simulink model "Copy_of_CoupledTanks_WCPS_v2_DoubleSD"  (Simulink 8.1)
settings: Solver=ode4  StartTime=0.0  StopTime=Tf  FixedStep=0.2  RelTol=1e-3
values from neighbouring files (symbols this model uses):
  A1 = 0.06    [Copy_of_CoupledTanks_WCPS_2_DoublePS.m]    (also in CoupledTanks_WCPS_2_DoublePS.m; DoublePlant_PS_INI3_RSSI74_1.mat; Wireless_74_Initial_98.mat)
  A2 = 0.3    [Copy_of_CoupledTanks_WCPS_2_DoublePS.m]    (also in CoupledTanks_WCPS_2_DoublePS.m; DoublePlant_PS_INI3_RSSI74_1.mat; Wireless_74_Initial_98.mat)
  alpha1 = 10    [Copy_of_CoupledTanks_WCPS_2_DoublePS.m]    (also in CoupledTanks_WCPS_2_DoublePS.m; DoublePlant_PS_INI3_RSSI74_1.mat; Wireless_74_Initial_98.mat)
  AR = 0.3    [Copy_of_CoupledTanks_WCPS_2_DoublePS.m]    (also in CoupledTanks_WCPS_2_DoublePS.m; DoublePlant_PS_INI3_RSSI74_1.mat; Wireless_74_Initial_98.mat)
  delta_t = 1    [Copy_of_CoupledTanks_WCPS_2_DoublePS.m]    (also in CoupledTanks_WCPS_2_DoublePS.m = 0.2; DoublePlant_PS_INI3_RSSI74_1.mat; Wireless_74_Initial_98.mat = 0.25)
  EMPeriod = 1    [Copy_of_CoupledTanks_WCPS_2_DoublePS.m]    (also in CoupledTanks_WCPS_2_DoublePS.m; DoublePlant_PS_INI3_RSSI74_1.mat; Wireless_74_Initial_98.mat = 8)
  g = 9.8    [Copy_of_CoupledTanks_WCPS_2_DoublePS.m]    (also in CoupledTanks_WCPS_2_DoublePS.m; DoublePlant_PS_INI3_RSSI74_1.mat; Wireless_74_Initial_98.mat)
  kd = 0    [Copy_of_CoupledTanks_WCPS_2_DoublePS.m]    (also in CoupledTanks_WCPS_2_DoublePS.m; DoublePlant_PS_INI3_RSSI74_1.mat; Wireless_74_Initial_98.mat)
  ki = 0.5    [Copy_of_CoupledTanks_WCPS_2_DoublePS.m]    (also in CoupledTanks_WCPS_2_DoublePS.m; DoublePlant_PS_INI3_RSSI74_1.mat; Wireless_74_Initial_98.mat)
  kp = 5    [Copy_of_CoupledTanks_WCPS_2_DoublePS.m]    (also in CoupledTanks_WCPS_2_DoublePS.m; DoublePlant_PS_INI3_RSSI74_1.mat; Wireless_74_Initial_98.mat)
  L1H = 9    [Copy_of_CoupledTanks_WCPS_2_DoublePS.m]    (also in CoupledTanks_WCPS_2_DoublePS.m = 90; DoublePlant_PS_INI3_RSSI74_1.mat; Wireless_74_Initial_98.mat)
  L1ini = 9    [Copy_of_CoupledTanks_WCPS_2_DoublePS.m]    (also in CoupledTanks_WCPS_2_DoublePS.m; DoublePlant_PS_INI3_RSSI74_1.mat; Wireless_74_Initial_98.mat = 8.14638203104)
  L1up = 10    [Copy_of_CoupledTanks_WCPS_2_DoublePS.m]    (also in CoupledTanks_WCPS_2_DoublePS.m; DoublePlant_PS_INI3_RSSI74_1.mat; Wireless_74_Initial_98.mat)
  L2H = 11.5    [Copy_of_CoupledTanks_WCPS_2_DoublePS.m]    (also in CoupledTanks_WCPS_2_DoublePS.m = 115; DoublePlant_PS_INI3_RSSI74_1.mat; Wireless_74_Initial_98.mat)
  L2ini = 9.15    [Copy_of_CoupledTanks_WCPS_2_DoublePS.m]    (also in CoupledTanks_WCPS_2_DoublePS.m; DoublePlant_PS_INI3_RSSI74_1.mat; Wireless_74_Initial_98.mat = 6.34545311751)
  L2sp = 11.05    [Copy_of_CoupledTanks_WCPS_2_DoublePS.m]    (also in CoupledTanks_WCPS_2_DoublePS.m; DoublePlant_PS_INI3_RSSI74_1.mat; Wireless_74_Initial_98.mat)
  L2up = 13    [Copy_of_CoupledTanks_WCPS_2_DoublePS.m]    (also in CoupledTanks_WCPS_2_DoublePS.m; DoublePlant_PS_INI3_RSSI74_1.mat; Wireless_74_Initial_98.mat)
  LRdown = 0    [Copy_of_CoupledTanks_WCPS_2_DoublePS.m]    (also in CoupledTanks_WCPS_2_DoublePS.m; DoublePlant_PS_INI3_RSSI74_1.mat; Wireless_74_Initial_98.mat)
  LRH = 5.7    [Copy_of_CoupledTanks_WCPS_2_DoublePS.m]    (also in CoupledTanks_WCPS_2_DoublePS.m = 57; DoublePlant_PS_INI3_RSSI74_1.mat; Wireless_74_Initial_98.mat)
  LRini = 5.65    [Copy_of_CoupledTanks_WCPS_2_DoublePS.m]    (also in CoupledTanks_WCPS_2_DoublePS.m; DoublePlant_PS_INI3_RSSI74_1.mat; Wireless_74_Initial_98.mat = 4.28399951136)
  LRL = 0.2    [Copy_of_CoupledTanks_WCPS_2_DoublePS.m]    (also in CoupledTanks_WCPS_2_DoublePS.m = 0; DoublePlant_PS_INI3_RSSI74_1.mat; Wireless_74_Initial_98.mat)
  LRup = 9    [Copy_of_CoupledTanks_WCPS_2_DoublePS.m]    (also in CoupledTanks_WCPS_2_DoublePS.m; DoublePlant_PS_INI3_RSSI74_1.mat; Wireless_74_Initial_98.mat)
  p12 = 1    [Copy_of_CoupledTanks_WCPS_2_DoublePS.m]    (also in CoupledTanks_WCPS_2_DoublePS.m; DoublePlant_PS_INI3_RSSI74_1.mat; Wireless_74_Initial_98.mat)
  p22 = 1    [Copy_of_CoupledTanks_WCPS_2_DoublePS.m]    (also in CoupledTanks_WCPS_2_DoublePS.m; DoublePlant_PS_INI3_RSSI74_1.mat; Wireless_74_Initial_98.mat)
  p2tap = 1    [Copy_of_CoupledTanks_WCPS_2_DoublePS.m]    (also in CoupledTanks_WCPS_2_DoublePS.m; DoublePlant_PS_INI3_RSSI74_1.mat; Wireless_74_Initial_98.mat)
  PumpMAX = 60    [Copy_of_CoupledTanks_WCPS_2_DoublePS.m]    (also in CoupledTanks_WCPS_2_DoublePS.m; DoublePlant_PS_INI3_RSSI74_1.mat; Wireless_74_Initial_98.mat)
  R1 = 0.0005    [Copy_of_CoupledTanks_WCPS_2_DoublePS.m]    (also in CoupledTanks_WCPS_2_DoublePS.m; DoublePlant_PS_INI3_RSSI74_1.mat; Wireless_74_Initial_98.mat)
  R1tap = 0.001    [Copy_of_CoupledTanks_WCPS_2_DoublePS.m]    (also in CoupledTanks_WCPS_2_DoublePS.m; DoublePlant_PS_INI3_RSSI74_1.mat; Wireless_74_Initial_98.mat)
  R2 = 0.001    [Copy_of_CoupledTanks_WCPS_2_DoublePS.m]    (also in CoupledTanks_WCPS_2_DoublePS.m; DoublePlant_PS_INI3_RSSI74_1.mat; Wireless_74_Initial_98.mat)
  rho = 1000    [Copy_of_CoupledTanks_WCPS_2_DoublePS.m]    (also in CoupledTanks_WCPS_2_DoublePS.m; DoublePlant_PS_INI3_RSSI74_1.mat; Wireless_74_Initial_98.mat)
settings Model: Creator=Rhine  LastModifiedBy=sywxh2012
settings DebuggingCC: MultiTaskDSMMsg=none  MultiTaskRateTransMsg=warning

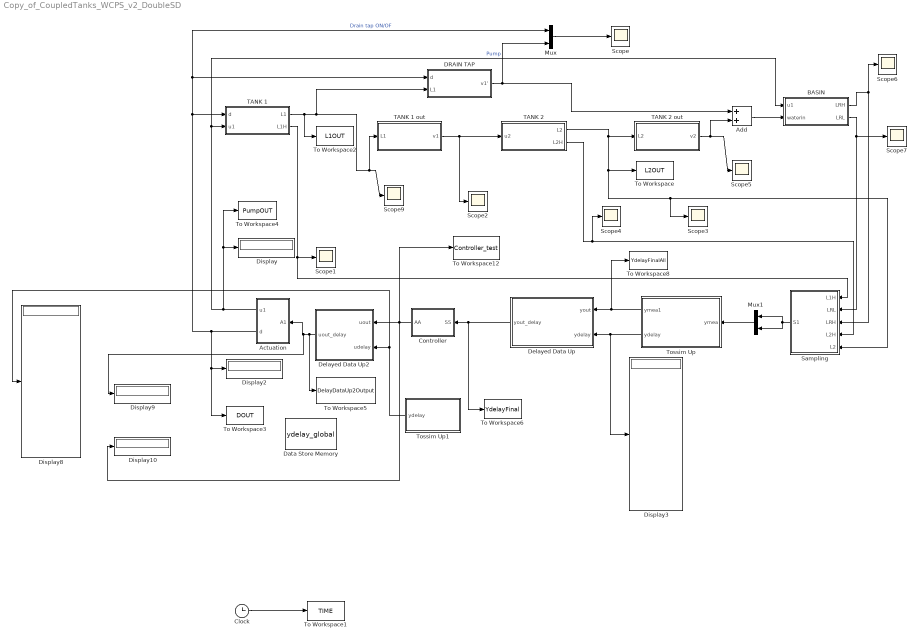
== system Copy_of_CoupledTanks_WCPS_v2_DoubleSD ==
  Actuation : Subsystem
  Add : Sum
  BASIN : Subsystem
  Clock : Clock
  Controller : Subsystem
  DRAIN TAP : Subsystem
  Data Store Memory : DataStoreMemory  DataStoreName=ydelay_global  ReadBeforeWriteMsg=warning  WriteAfterWriteMsg=warning  WriteAfterReadMsg=warning  InitialValue=[1; 1; 1; 1; 1; 1; 1; 1; 1; 1; 1; 1; 1; 1; 1]  OutDataTypeStr=uint32
  Delayed Data Up : MATLAB Function  TreatAsAtomicUnit=on
  Delayed Data Up2 : MATLAB Function  TreatAsAtomicUnit=on
  Display{,2..3,8..10} (6 alike) : Display
  Mux : Mux  Inputs=2
  Mux1 : Mux  Inputs=2
  Sampling : Subsystem
  Scope{,1..7,9} (9 alike) : Scope
      Scope2 settings: SaveName=ScopeData2
      Scope3 settings: SaveName=ScopeData15
      Scope4 settings: SaveName=ScopeData4
      Scope5 settings: SaveName=ScopeData5
      Scope6 settings: SaveName=ScopeData7
      Scope7 settings: SaveName=ScopeData8
      Scope9 settings: YMin=7.45104  YMax=8.23536  SaveName=ScopeData10
  TANK 1 : Subsystem
  TANK 1 out : Subsystem
  TANK 2 : Subsystem
  TANK 2 out : Subsystem
  To Workspace : ToWorkspace  VariableName=L2OUT  SampleTime=-1
  To Workspace1 : ToWorkspace  VariableName=TIME  SampleTime=-1
  To Workspace12 : ToWorkspace  VariableName=Controller_test  SampleTime=-1
  To Workspace2 : ToWorkspace  VariableName=L1OUT  SampleTime=-1
  To Workspace3 : ToWorkspace  VariableName=DOUT  SampleTime=-1
  To Workspace4 : ToWorkspace  VariableName=PumpOUT  SampleTime=-1
  To Workspace5 : ToWorkspace  VariableName=DelayDataUp2Output  SampleTime=-1
  To Workspace6 : ToWorkspace  VariableName=YdelayFinal  SampleTime=-1
  To Workspace8 : ToWorkspace  VariableName=YdelayFinalAll  SampleTime=-1
  Tossim Up : MATLAB Function  TreatAsAtomicUnit=on
  Tossim Up1 : MATLAB Function  TreatAsAtomicUnit=on
  wires:
  TANK 1/1(L1) -> DRAIN TAP/2(L1), TANK 1 out/1(L1), Scope9/1, To Workspace2/1
  TANK 2/1(L2) -> TANK 2 out/1(L2), To Workspace/1, Scope3/1, Sampling/5(L2)
  DRAIN TAP/1(v1') -> Add/1, Mux/2
  TANK 2 out/1(v2) -> Scope5/1, Add/2
  TANK 1/2(L1H) -> Scope1/1, Sampling/1(L1H)
  TANK 1 out/1(v1) -> TANK 2/1(u2), Scope2/1
  TANK 2/2(L2H) -> Scope4/1, Sampling/4(L2H)
  Add/1 -> BASIN/2(waterin)
  BASIN/1(LRH) -> Scope6/1, Sampling/3(LRH)
  BASIN/2(LRL) -> Scope7/1, Sampling/2(LRL)
  Actuation/1(u1) -> Display/1, To Workspace4/1, TANK 1/2(u1), BASIN/1(u1)  "Pump"
  Actuation/2(d) -> TANK 1/1(d), DRAIN TAP/1(d), Mux/1, Display2/1, To Workspace3/1  "Drain tap ON/OF"
  Clock/1 -> To Workspace1/1
  Mux/1 -> Scope/1
  Tossim Up/1(ymea1) -> Delayed Data Up/1(yout), To Workspace8/1
  Tossim Up/2(ydelay) -> Display3/1, Delayed Data Up/2(ydelay)
  Sampling/1(S1) -> Mux1/2, Mux1/1
  Mux1/1 -> Tossim Up/1(ymea)
  Controller/1(AA) -> To Workspace12/1, Display10/1, Delayed Data Up2/1(uout)
  Delayed Data Up2/1(uout_delay) -> To Workspace5/1, Display9/1, Actuation/1(A1)
  Tossim Up1/1(ydelay) -> Display8/1, Delayed Data Up2/2(udelay)
  Delayed Data Up/1(yout_delay) -> To Workspace6/1, Controller/1(SS)

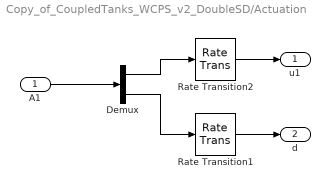
== system Copy_of_CoupledTanks_WCPS_v2_DoubleSD/Actuation ==
  A1 : Inport
  Demux : Demux  Outputs=2
  Rate Transition1 : RateTransition  OutPortSampleTime=delta_t
  Rate Transition2 : RateTransition  OutPortSampleTime=delta_t
  u1 : Outport
  d : Outport  Port=2
  wires:
  A1/1 -> Demux/1
  Rate Transition2/1 -> u1/1
  Rate Transition1/1 -> d/1
  Demux/1 -> Rate Transition2/1
  Demux/2 -> Rate Transition1/1

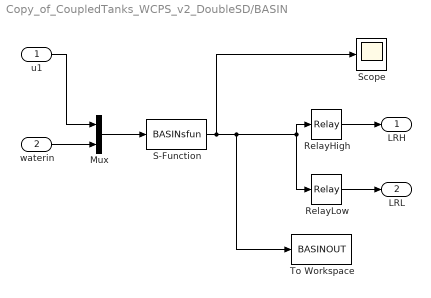
== system Copy_of_CoupledTanks_WCPS_v2_DoubleSD/BASIN ==
  u1 : Inport
  waterin : Inport  Port=2
  Mux : Mux  Inputs=2
  RelayHigh : Relay  OnSwitchValue=LRH  OffSwitchValue=LRH
  RelayLow : Relay  OnSwitchValue=LRL  OffSwitchValue=LRL  OnOutputValue=0  OffOutputValue=1
  S-Function : S-Function  FunctionName=BASINsfun  Parameters=alpha1,AR,LRup,LRdown,rho,LRini  EnableBusSupport=off
  Scope : Scope
      settings: SaveName=ScopeData6
  To Workspace : ToWorkspace  VariableName=BASINOUT  SampleTime=-1
  LRH : Outport
  LRL : Outport  Port=2
  wires:
  RelayLow/1 -> LRL/1
  RelayHigh/1 -> LRH/1
  S-Function/1 -> RelayHigh/1, RelayLow/1, To Workspace/1, Scope/1
  u1/1 -> Mux/1
  waterin/1 -> Mux/2
  Mux/1 -> S-Function/1

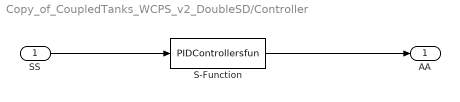
== system Copy_of_CoupledTanks_WCPS_v2_DoubleSD/Controller ==
  SS : Inport
  S-Function : S-Function  FunctionName=PIDControllersfun  Parameters=L2sp,kp,ki,kd,PumpMAX,delta_t,EMPeriod,L2ini  EnableBusSupport=off
  AA : Outport
  wires:
  SS/1 -> S-Function/1
  S-Function/1 -> AA/1

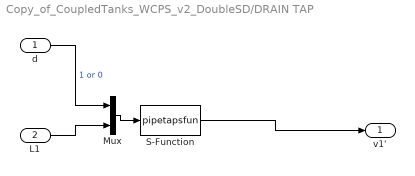
== system Copy_of_CoupledTanks_WCPS_v2_DoubleSD/DRAIN TAP ==
  d : Inport
  L1 : Inport  Port=2
  Mux : Mux  Inputs=2
  S-Function : S-Function  FunctionName=pipetapsfun  Parameters=rho,R1tap,p2tap,g  EnableBusSupport=off
  v1' : Outport
  wires:
  d/1 -> Mux/1  "1 or 0"
  L1/1 -> Mux/2
  Mux/1 -> S-Function/1
  S-Function/1 -> v1'/1

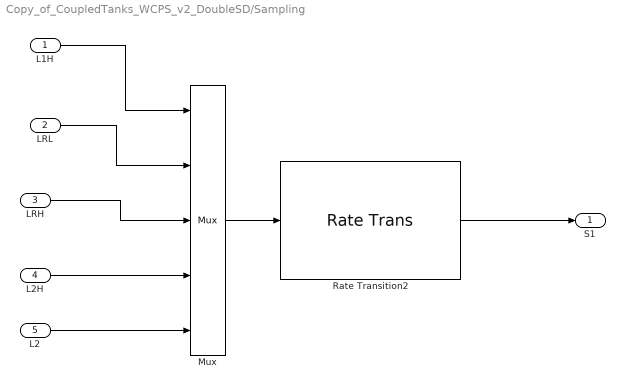
== system Copy_of_CoupledTanks_WCPS_v2_DoubleSD/Sampling ==
  L1H : Inport
  LRL : Inport  Port=2
  LRH : Inport  Port=3
  L2H : Inport  Port=4
  L2 : Inport  Port=5
  Mux : Mux  Inputs=5
  Rate Transition2 : RateTransition  OutPortSampleTime=delta_t
  S1 : Outport
  wires:
  Mux/1 -> Rate Transition2/1
  L1H/1 -> Mux/1
  LRL/1 -> Mux/2
  LRH/1 -> Mux/3
  L2H/1 -> Mux/4
  L2/1 -> Mux/5
  Rate Transition2/1 -> S1/1

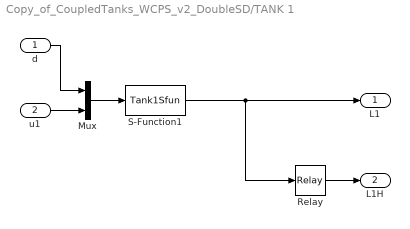
== system Copy_of_CoupledTanks_WCPS_v2_DoubleSD/TANK 1 ==
  d : Inport
  u1 : Inport  Port=2
  Mux : Mux  Inputs=2
  Relay : Relay  OnSwitchValue=L1H  OffSwitchValue=L1H
  S-Function1 : S-Function  FunctionName=Tank1Sfun  Parameters=A1,L1up,rho,alpha1,R1,p12,R1tap,p2tap,g,L1ini  EnableBusSupport=off
  L1 : Outport
  L1H : Outport  Port=2
  wires:
  Relay/1 -> L1H/1
  S-Function1/1 -> L1/1, Relay/1
  d/1 -> Mux/1
  u1/1 -> Mux/2
  Mux/1 -> S-Function1/1

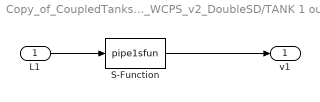
== system Copy_of_CoupledTanks_WCPS_v2_DoubleSD/TANK 1 out ==
  L1 : Inport
  S-Function : S-Function  FunctionName=pipe1sfun  Parameters=rho,R1,p12,g  EnableBusSupport=off
  v1 : Outport
  wires:
  L1/1 -> S-Function/1
  S-Function/1 -> v1/1

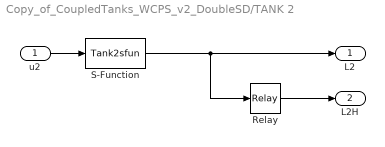
== system Copy_of_CoupledTanks_WCPS_v2_DoubleSD/TANK 2 ==
  u2 : Inport
  Relay : Relay  OnSwitchValue=L2H  OffSwitchValue=L2H
  S-Function : S-Function  FunctionName=Tank2sfun  Parameters=A2,L2up,rho,R2,p22,g,L2ini  EnableBusSupport=off
  L2 : Outport
  L2H : Outport  Port=2
  wires:
  Relay/1 -> L2H/1
  u2/1 -> S-Function/1
  S-Function/1 -> L2/1, Relay/1

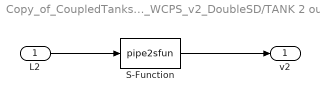
== system Copy_of_CoupledTanks_WCPS_v2_DoubleSD/TANK 2 out ==
  L2 : Inport
  S-Function : S-Function  FunctionName=pipe2sfun  Parameters=rho,R2,p22,g  EnableBusSupport=off
  v2 : Outport
  wires:
  L2/1 -> S-Function/1
  S-Function/1 -> v2/1

== matlab function Tossim Up ==
  data: ymea1 output double; ymea input double; ydelay output double; ydelay_global data_store_memory double
function [ymea1, ydelay]  = Tossim_block(ymea)
% Inputs:
% ymea: measurement from structure
% Outputs:
% ymea1: measurement output
% ydelay: delay traces
persistent delay1 % delay trace
persistent i  % count
persistent last_emergency_instance RetransCounter
global ydelay_global


% allow these matlab functions to be used in Embedded Matlab block
eml.extrinsic('python');
eml.extrinsic('num2str');
eml.extrinsic('str2num');
eml.extrinsic('delay_summary');
eml.extrinsic('disp');
eml.extrinsic('ps_aggregation');
eml.extrinsic('for');
eml.extrinsic('end');

if isempty(i)
    i = 0;
end

ydelay = [1 0 0 0 0 0 0 0 0 0 0 0 0 0 0]'; %No, delay of L1H, delay of L2H, delay of L2, delay of LRL, delay of LRH delay of L1H, delay of L2H, delay of L2, delay of LRL, delay of LRH
% call python to communicate with TOSSIM
emergency_instance=ymea'

%below created in iccps15
%call_count = 55; % number of slots + 1 for PS(i.e., number of client calls made + 1) per TDMA schedule, +1 to have full 53 slots executed
call_count = 49; % number of slots + 1 for Slote Stealing(i.e., number of client calls made + 1) per TDMA schedule, +1 to have full 53 slots executed

rssi = -74;%below is where we inject the senosor status into TOSSIM

[resultz] = ps_aggregation(call_count, rssi, emergency_instance);

end_to_end_delivery_result_aggregated = sum(resultz)
[delay] = delay_summary(end_to_end_delivery_result_aggregated);

delay

% assign delay
ydelay = delay';

last_emergency_instance=ymea';
delay1 = ydelay;
i = i+1;

ymea1 = [0 0 0 0 0 0 0 0 0 0]'; %two plants, 10 sensors
ymea1 = ymea;

for i_yg = 1:15
    ydelay_global(i_yg, 1) = ydelay(i_yg, 1);
end

% disp('Plant 1, TOSSIM Uplink Block, is called');

== matlab function Delayed Data Up ==
  data: yout input double; ydelay input double; yout_delay output double; structure parameter double
function yout_delay   = delay_block(yout,ydelay, structure)

% Inputs: 
% yout: measurements output
% ydelay: delay traces
% structure: other necessary information 
% Inputs: 
% yout: measurements output
% ydelay: delay traces

% Outputs:
% yout_delay: delayed measurements output for controller
persistent  i yin_d 
persistent yin delay yin_all num
eml.extrinsic('disp');

sennum=5;  %number of the sensors
step_count=100000; %step_count

% initialize parameters
if isempty(yin)
    i = structure.i;
    yin = structure.yin;
    yin_d = structure.yin_d; 
    yin_all = zeros(step_count+1,5); %zeros (step count, sensor number)
    
    delay = zeros(1,5+1);         %initialized
    delay = ydelay';
    
    num = 0;
end

num = num+1;   

%get delay information 
delay=zeros(1,5+1); 
delay=ydelay';

%get value from "yout" input
for kk = 1:5
    yin_all(num,kk) = yout(kk);
end    
    
%generate output value according to delay    
for j=1:5
    if delay(1,j+1)~=88
        yin(j) = yin_all(num,j);  %packet receive
    else
        if num>1 
%             yin(j)=0;  %if lost, set it to zero
             yin(j)=yin_all(num-1,j); %if lost, set it to previous value
             yin_all(num,j)=yin_all(num-1,j);
        end        
    end
end

yin_d = yin';
yout_delay = yin_d;

i = i+1;

== matlab function Delayed Data Up2 ==
  data: uout input double; uout_delay output double; udelay input double
function uout_delay   = delay_blocku(uout,udelay)

% Inputs: 
% yout: measurements output
% udelay: delay traces
% structure: other necessary information 
% Inputs: 
% yout: measurements output
% udelay: delay traces

% Outputs:
% yout_delay: delayed measurements output for controller

persistent  i uin_d 
persistent uin delay uin_all numAct
eml.extrinsic('disp');

actnum=2;  %number of the actuators
step_count=100000; %step_count

% initialize parameters
if isempty(uin)
    i = 0;
    uin = [0 0];
    uin_d = [0 0]'; 
    uin_all = zeros(step_count+1,2); %zeros (step count, sensor number)
    
    delay = zeros(1,14+1);         %initialized
    delay = udelay';
    
    numAct = 0;
end


%udelay=[1 1 1 1 1 1]';

numAct = numAct+1;

%get delay information 
delay=zeros(1,14+1); 
delay=udelay';

%get value from "yout" input
for kk = 1:2
    uin_all(numAct,kk) = uout(kk);
end    
    
%generate output value according to delay    
for j=1:2
    if delay(1,j+11)~=88
        uin(j) = uin_all(numAct,j);  %packet receive
    else
        if numAct>1 
%             yin(j)=0;  %if lost, set it to zero
             uin(j)=uin_all(numAct-1,j); %if lost, set it to previous value
             uin_all(numAct,j)=uin_all(numAct-1,j);
        end        
    end
end


uin_d = uin';

uout_delay = uin_d;

i = i+1;

% disp('downlink data block called:')
% udelay(12:13, 1)'
% uout_delay'
% 

%yout_delay;
disp('yout_delay');
%disp('yout_delay');
%disp('data usage 2 i')
disp(i)

% disp('numAct')
% numAct

== matlab function Tossim Up1 ==
  data: ydelay output double; ydelay_global data_store_memory double
function ydelay   = Tossim_block
% Inputs:
% ymea: measurement from structure
% Outputs:
% ymea1: measurement output
% ydelay: delay traces
persistent delay1 % delay trace
persistent i  % count
persistent last_emergency_instance RetransCounter

% allow these matlab functions to be used in Embedded Matlab block
eml.extrinsic('python');
eml.extrinsic('num2str');
eml.extrinsic('delay_summary');
eml.extrinsic('disp');
if isempty(i)
    i = 0;
end
ymea=[1 1 1 1 1]';

%ydelay = [1 0 0 0 0 0 0 0]'; %No, delay of L1H,  delay of LRL, delay of LRH delay of L2H, delay of L2, delay of pump, delay of drain

ydelay = [1 0 0 0 0 0 0 0 0 0 0 0 0 0 0]'; %No, delay of L1H, delay of L2H, delay of L2, delay of LRL, delay of LRH£¬delay of L1H, delay of L2H, delay of L2, delay of LRL, delay of LRH
% call python to communicate with TOSSIM
emergency_instance=ymea';

%belwo created in iccps15
ydelay = ones (15, 1);

global ydelay_global
for i_tb1 = 1:15
    ydelay(i_tb1, 1) = ydelay_global(i_tb1, 1);
end

delay1 = ydelay;
i = i+1;

ymea1 = [0 0 0 0 0]';
ymea1 = ymea;
